simulink library "tetherBuoyancyAndWeightNGreater2_ul"  (R2018b)
settings: Solver=VariableStepAuto  StartTime=0.0  StopTime=10.0  RelTol=1e-3
values from neighbouring files (symbols this model uses):
  dia_t = 0.1    [tetherBuoyancyAndWeight.m]    (also in tetherBuoyancyAndWeight_ts.m)
  g = 9.81    [tetherBuoyancyAndWeight_ts.m]
  N = 4    [tetherBuoyancyAndWeight.m]    (also in tetherBuoyancyAndWeight_ts.m)
  rho_fluid = 1000    [tetherBuoyancyAndWeight.m]    (also in tetherBuoyancyAndWeight_ts.m)
  rho_tether = 900    [tetherBuoyancyAndWeight.m]    (also in tetherBuoyancyAndWeight_ts.m)
libraries: simulink x1, cylinderVolume_ul x1
settings Model: Creator=asiddiq2  LastModifiedBy=asiddiq2

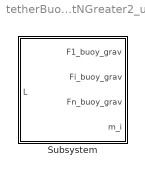
== system tetherBuoyancyAndWeightNGreater2_ul ==
  Subsystem : Subsystem  mask{N=N, dia_t=dia_t, rho_fluid=rho_fluid, rho_tether=rho_tether, g=g}
      mask prompts: N "Number of nodes (N>=2)"; dia_t "Tether diameter (m)"; rho_fluid "Fluid density (kg/m^3)"; rho_tether "Tether density (kg/m^3)"; g "Gravitational acceleration (m/s^2)"

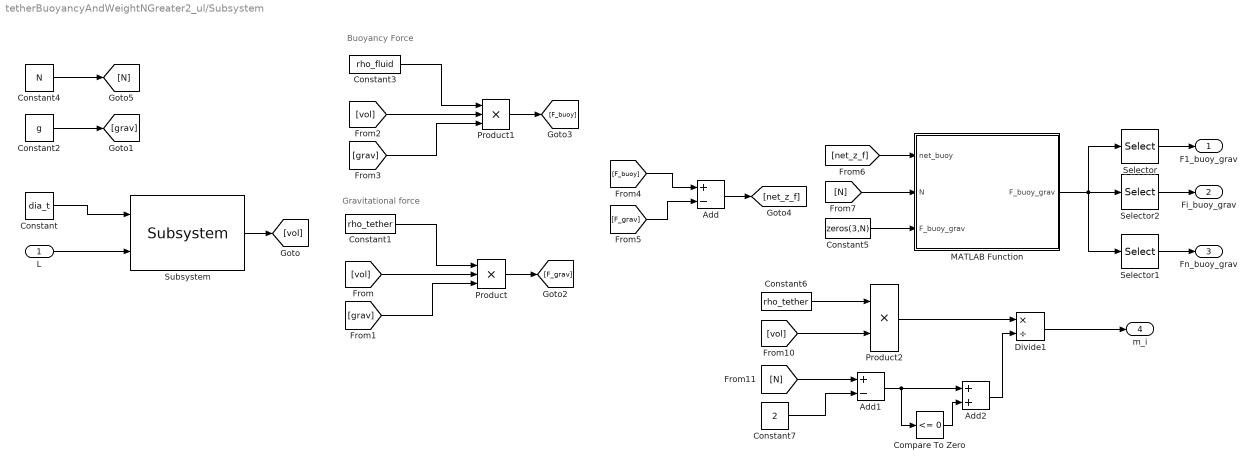
== system tetherBuoyancyAndWeightNGreater2_ul/Subsystem ==
  note: Buoyancy Force
  note: Gravitational force
  L : Inport
  Add : Sum  Inputs=+-
  Add1 : Sum  Inputs=+-
  Add2 : Sum
  Compare To Zero : simulink/Logic and Bit Operations/Compare To Zero  relop=<=  OutDataTypeStr=boolean
  Constant : Constant  Value=dia_t
  Constant1 : Constant  Value=rho_tether
  Constant2 : Constant  Value=g
  Constant3 : Constant  Value=rho_fluid
  Constant4 : Constant  Value=N
  Constant5 : Constant  Value=zeros(3,N)
  Constant6 : Constant  Value=rho_tether
  Constant7 : Constant  Value=2
  Divide1 : Product  Inputs=*/
  MATLAB Function : MATLAB Function  TreatAsAtomicUnit=on
  Product : Product  Inputs=3
  Product1 : Product  Inputs=3
  Product2 : Product
  Selector : Selector  NumberOfDimensions=2  InputPortWidth=3  IndexOptions=Select all,Index vector (dialog)  Indices=[1 3],1  OutputSizes=1,1
  Selector1 : Selector  NumberOfDimensions=2  InputPortWidth=3  IndexOptions=Select all,Index vector (dialog)  Indices=[1 3],N  OutputSizes=1,1
  Selector2 : Selector  NumberOfDimensions=2  InputPortWidth=3  IndexOptions=Select all,Index vector (dialog)  Indices=[1 3],[2:N-1]  OutputSizes=1,1
  Subsystem : cylinderVolume_ul/Subsystem  SystemSampleTime=-1
  F1_buoy_grav : Outport
  Fi_buoy_grav : Outport  Port=2
  Fn_buoy_grav : Outport  Port=3
  m_i : Outport  Port=4
  wires:
  L/1 -> Subsystem/2
  Constant/1 -> Subsystem/1
  Subsystem/1 -> [vol]
  Constant2/1 -> [grav]
  Constant1/1 -> Product/1
  [vol] -> Product/2
  [grav] -> Product/3
  Product/1 -> [F_grav]
  [grav] -> Product1/3
  Constant3/1 -> Product1/1
  [vol] -> Product1/2
  Product1/1 -> [F_buoy]
  [F_buoy] -> Add/1
  [F_grav] -> Add/2
  Add/1 -> [net_z_f]
  [net_z_f] -> MATLAB Function/1(net_buoy)
  Constant4/1 -> [N]
  [N] -> MATLAB Function/2(N)
  Constant5/1 -> MATLAB Function/3("F_buoy_grav ")
  [vol] -> Product2/2
  Constant6/1 -> Product2/1
  Product2/1 -> Divide1/1
  Divide1/1 -> m_i/1
  [N] -> Add1/1
  Add1/1 -> Add2/1, Compare To Zero/1
  Constant7/1 -> Add1/2
  Compare To Zero/1 -> Add2/2
  Add2/1 -> Divide1/2
  Selector/1 -> F1_buoy_grav/1
  Selector1/1 -> Fn_buoy_grav/1
  MATLAB Function/1(F_buoy_grav) -> Selector1/1, Selector2/1, Selector/1
  Selector2/1 -> Fi_buoy_grav/1

== matlab function tetherBuoyancyAndWeightNGreater2_ul/Subsystem/MATLAB Function ==
  data: net_buoy input; F_buoy_grav output; N input; F_buoy_grav input
function F_buoy_grav = fcn(net_buoy,N,F_buoy_grav)

for i = 1:N
    if i == 1
        F_buoy_grav(:,i) = zeros(3,1);
    elseif i>1 && i<N
        F_buoy_grav(:,i) = net_buoy/(N-2)*[0; 0; 1];
    elseif i == N
        F_buoy_grav(:,i) = zeros(3,1);
    end
    
end

end
